simulink model "room_temp"  (R2018a)
settings: Solver=FixedStepDiscrete  StartTime=0.0  StopTime=10.0  RelTol=1e-3
libraries: simulink x1
settings Model: Creator=Admin  LastModifiedBy=Admin
settings OptimizationCC: DefaultParameterBehavior=Inlined  EnhancedBackFolding=on  PassReuseOutputArgsAs=Individual arguments  OptimizeBlockOrder=speed  DifferentSizesBufferReuse=on  OptimizationCustomize=off
settings DebuggingCC: ParameterTunabilityLossMsg=error
settings SFSimCC: MATLABDynamicMemAlloc=off
settings RTWCC: SystemTargetFile=ert.tlc  GenCodeOnly=on  TemplateMakefile=ert_default_tmf  GenerateReport=on  IncludeHyperlinkInReport=on  LaunchReport=on  GenerateTraceInfo=on  GenerateTraceReport=on  GenerateTraceReportSl=on  GenerateTraceReportSf=on  GenerateTraceReportEml=on
settings CodeAppCC: ForceParamTrailComments=on  IgnoreCustomStorageClasses=off  OperatorAnnotations=on  SimulinkDataObjDesc=on  SFDataObjDesc=on  InsertBlockDesc=on
settings ERTTargetCC: TargetLangStandard=C99 (ISO)  GenerateSampleERTMain=on  InlinedParameterPlacement=NonHierarchical  ERTCustomFileTemplate=example_file_process.tlc

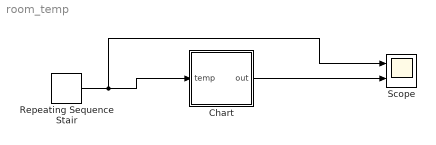
== system room_temp ==
  Chart : Stateflow chart  TreatAsAtomicUnit=on
  Repeating Sequence Stair : simulink/Sources/Repeating Sequence Stair  OutValues=[20 21 22 23 24 25 26 27 28 29 30].'  tsamp=-1  OutMin=[]  OutMax=[]  OutDataTypeStr=double  OutputDataTypeScalingMode=double  OutDataType=fixdt(0,8)  ConRadixGroup=Best Precision: Vector-wise  OutScaling=2^-12
  Scope : Scope  NumInputPorts=2
  wires:
  Chart/1(out) -> Scope/2
  Repeating Sequence Stair/1 -> Scope/1, Chart/1(temp)

== stateflow chart room_temp/Chart ==
  state off
    en:
    out=0;
  state cooler
    en:
    out=-1;
  state Heater
    en:
    out=1;
  (default) -> (junction 53)
  (junction 53) -> cooler [order 4]
  (junction 53) -> (junction 58) [order 2] : [temp>=23 && temp<=27]
  (junction 53) -> (junction 59) [order 1] : [temp>27]
  (junction 58) -> off
  (junction 53) -> Heater [order 3] : [temp<23]
  (junction 59) -> cooler
  off -> cooler [order 1] : [temp>27]
  cooler -> off [order 2] : [temp>=23 && temp<=27]
  cooler -> Heater [order 1] : [temp<23]
  Heater -> cooler [order 2] : [temp>27]
  off -> Heater [order 2] : [temp<23]
  Heater -> off [order 1] : [temp>=23 && temp<=27]
  data: out output; temp input
